simulink model "a_b_x_y"  (R2023b)
settings: Solver=FixedStepAuto  StartTime=0.0  StopTime=inf  RelTol=1e-3  EnableMultiTasking=on
model workspace (MAT data in the model file):
  G = 2001
libraries: rpi_blkst x2
settings Model: ExtModeTrigDuration=2  Creator=yabde  LastModifiedBy=yacine-a
settings SolverCC: PositivePriorityOrder=on
settings OptimizationCC: EnhancedBackFolding=on  PassReuseOutputArgsAs=Individual arguments  ZeroExternalMemoryAtStartup=off  ZeroInternalMemoryAtStartup=off  MaxStackSize=64  OptimizeBlockOrder=speed  DifferentSizesBufferReuse=on  OptimizationCustomize=off  EfficientTunableParamExpr=on
settings DebuggingCC: ParameterTunabilityLossMsg=error
settings HardwareCC: ProdBitPerLong=64  ProdLargestAtomicInteger=LongLong  ProdLargestAtomicFloat=Double  ProdLongLongMode=on  ProdHWDeviceType=ARM Compatible->ARM 64-bit (LP64)
settings RTWCC: Description=Embedded Coder  SystemTargetFile=ert.tlc  HardwareBoard=Raspberry Pi (64bit)  TLCOptions="-aInlineSetEventsForThisBaseRateFcn=TLC_FALSE -aSuppressMultiTaskScheduler=TLC_FALSE  -aRateBasedStepFcn=0"  TemplateMakefile=ert_default_tmf  Toolchain=GNU GCC Embedded Linux  BuildConfiguration=Faster Runs
settings CodeAppCC: ForceParamTrailComments=on  IgnoreCustomStorageClasses=off  OperatorAnnotations=on  SimulinkDataObjDesc=on  SFDataObjDesc=on  InsertBlockDesc=on
settings ERTTargetCC: SupportVariableSizeSignals=on  ExtModeTransport=2  ExtModeStaticAlloc=on  ExtModeMexFile=ext_xcp  ExtModeIntrfLevel=Level2 - Open

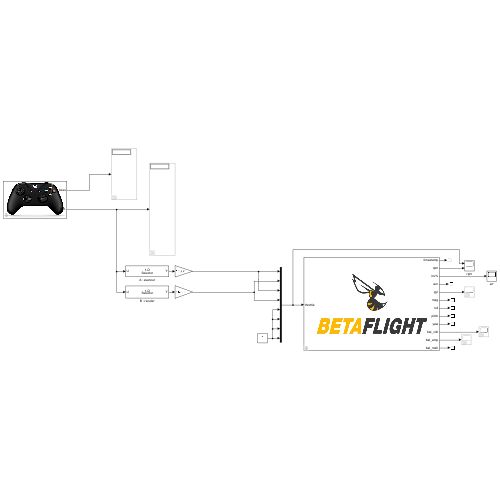
[thumbnail: Simulink's stored preview of the top-level diagram]
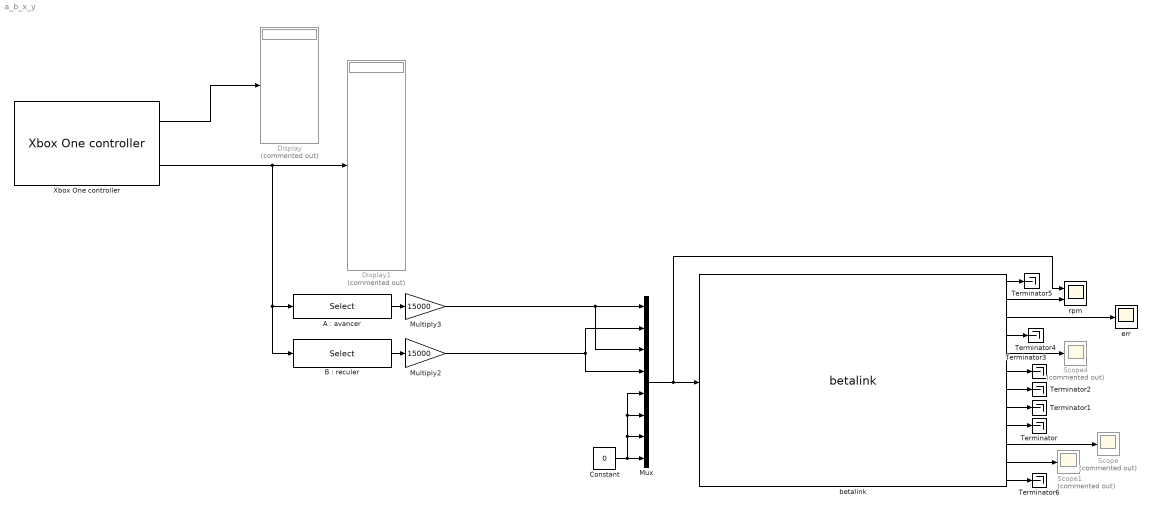
== system a_b_x_y ==
  "A : avancer" : Selector  IndexOptions=Index vector (dialog)  Indices=1  OutputSizes=1  RuntimeRangeChecks=on
  "B : reculer" : Selector  IndexOptions=Index vector (dialog)  Indices=2  OutputSizes=1  RuntimeRangeChecks=on
  Constant : Constant  Value=0
  Display : Display  Commented=on
  Display1 : Display  Commented=on
  Multiply2 : Gain  Gain=15000
  Multiply3 : Gain  Gain=15000
  Mux : Mux  Inputs=8
  Scope : Scope  Commented=on
  Scope1 : Scope  Commented=on
  Scope4 : Scope  Commented=on
  Terminator{,1..6} (7 alike) : Terminator
  Xbox One controller : rpi_blkst/Xbox One controller  rpi_mask_ID=0  rpi_mask_Ts=0.01
      settings: SourceProductName=RPI Blockset
  betalink : rpi_blkst/betalink  rpi_mask_usb_serial_number=1042260556  rpi_mask_Ts=0.01
      settings: SourceProductName=RPI Blockset
  err : Scope
  rpm : Scope  NumInputPorts=2
  wires:
  Mux/1 -> betalink/1, rpm/1
  Constant/1 -> Mux/5, Mux/6, Mux/7, Mux/8
  betalink/10 -> Scope/1
  betalink/11 -> Scope1/1
  betalink/2 -> rpm/2
  betalink/3 -> err/1
  betalink/5 -> Scope4/1
  betalink/9 -> Terminator/1
  betalink/8 -> Terminator1/1
  betalink/7 -> Terminator2/1
  betalink/6 -> Terminator3/1
  betalink/4 -> Terminator4/1
  betalink/12 -> Terminator6/1
  Xbox One controller/2 -> "B : reculer"/1, "A : avancer"/1, Display1/1
  Xbox One controller/1 -> Display/1
  betalink/1 -> Terminator5/1
  "A : avancer"/1 -> Multiply3/1
  "B : reculer"/1 -> Multiply2/1
  Multiply3/1 -> Mux/3, Mux/1
  Multiply2/1 -> Mux/2, Mux/4
